simulink model "GPSReadLog"  (Simulink 6.6)
settings: Solver=FixedStepDiscrete  StartTime=0.0  StopTime=10.0  FixedStep=0.01  RelTol=1e-3
InitFcn:
  | initGPS
undefined symbols (not defined in the file or in its folder): gpsInit, gpsParse, gpsRead, gpsSeparate, logData, loggerInit, spiSend, u1, uartInit, y1
libraries: dsPICdrivers x15, simulink x1, xpclib x1
settings Model: Creator=ASL_Lab  LastModifiedBy=ASL_Lab  ProdHWDeviceType=16-bit Generic
settings OptimizationCC: InlineParams=on  OptimizeModelRefInitCode=on  LifeSpan=1
settings HardwareCC: ProdBitPerInt=16  ProdEndianess=LittleEndian  ProdWordSize=16  ProdHWDeviceType=16-bit Generic  TargetHWDeviceType=32-bit Generic
settings RTWCC: SystemTargetFile=dspic.tlc  TemplateMakefile=dspic_pic30_gcc.tmf  PostCodeGenCommand=dsPIC_Compile()  Description=Embedded Target for Microchip dsPIC (real-time)  GenerateReport=on  ProcessScript=dspic_make_rtw_hook  IncludeHyperlinkInReport=on  LaunchReport=on
settings RTWCC: CustomSource=|
  | clib\circBuffer.c
  | clib\gpsParse.c
  | clib\gpsSplit.c
  | clib\sbrk.c
  | clib\bufferedUART.c
  | clib\dataLogger.c
settings CodeAppCC: IgnoreCustomStorageClasses=off
settings STFCustomTargetCC: TargetFcnLib=ansi_tfl_tmw.mat  GenFloatMathFcnCalls=ANSI_C  ModelReferenceCompliant=off  IncludeMdlTerminateFcn=off  CombineOutputUpdateFcns=on  SuppressErrorStatus=on  ERTCustomFileBanners=on  SupportContinuousTime=off  SupportNonInlinedSFcns=off  SystemTargetFile=dspic.tlc
settings ERTTargetCC: TargetFcnLib=ansi_tfl_tmw.mat  GenFloatMathFcnCalls=ANSI_C  ModelReferenceCompliant=off  IncludeMdlTerminateFcn=off  SuppressErrorStatus=on  ModelStepFunctionPrototypeControlCompliant=off  ExtModeMexFile=noextcomm  InlinedParameterPlacement=NonHierarchical  ERTSrcFileBannerTemplate=dsPIC_code_template.cgt  ERTHdrFileBannerTemplate=dsPIC_code_template.cgt  ERTDataSrcFileTemplate=dsPIC_code_template.cgt  ERTDataHdrFileTemplate=dsPIC_code_template.cgt  ERTCustomFileTemplate=dsPIC_main.tlc
settings CustomProperty: DataType=string  Value=C:\PROGRA~1\MATLAB\R2007a\rtw\bin\win32\gmake

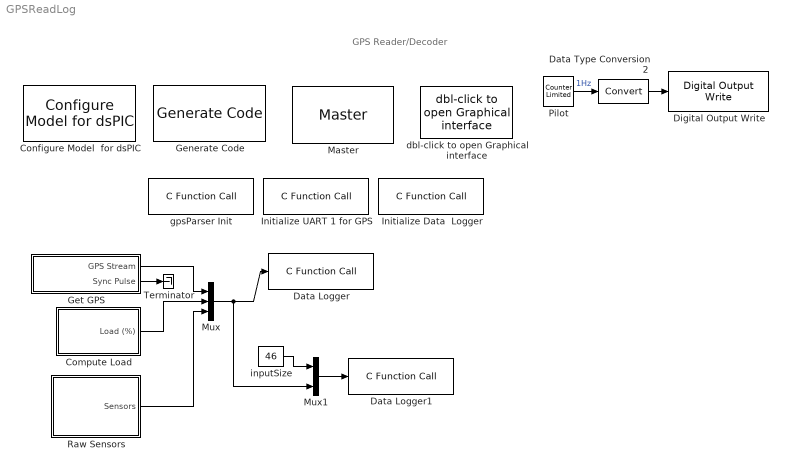
== system GPSReadLog ==
  note: GPS Reader/Decoder
  Compute Load : Subsystem
  Configure Model  for dsPIC : dsPICdrivers/Simulink Configuration/Configure Model  for dsPIC
  Data Logger : dsPICdrivers/OTHERS/C Function Call  Tag=dsPIC_dsPIC_CFunctionCall  fctName='logData'  INPUT_SIZE=46  INPUT1=uint8  INPUT2=--  INPUT3=--  OUTPUT_SIZE=1  OUTPUT1=--  SampleTime=-1  InputType=[ 2 ]  OutputType=[ ]  FctDeclaration=extern void logData(uint8_T* u1);  FctCall=logData(*%u1);  OrderingInOutPopup=None
  Data Logger1 : dsPICdrivers/OTHERS/C Function Call  Tag=dsPIC_dsPIC_CFunctionCall  fctName='spiSend'  INPUT_SIZE=47  INPUT1=uint8  INPUT2=--  INPUT3=--  OUTPUT_SIZE=1  OUTPUT1=--  SampleTime=-1  InputType=[ 2 ]  OutputType=[ ]  FctDeclaration=extern void spiSend(uint8_T* u1);  FctCall=spiSend(*%u1);  OrderingInOutPopup=None
  Data Type Conversion2 : DataTypeConversion  OutDataTypeMode=boolean
  Digital Output Write : dsPICdrivers/Digital I//O/Digital Output Write  Tag=dsPIC_Digital_Output  Priority=5  PORT=G  Pin=[ 14]  Simultaneous=off  OrderingInOutPopup=None
  Generate Code : dsPICdrivers/Simulink Configuration/Generate Code
  Get GPS : Subsystem
  Initialize Data  Logger : dsPICdrivers/OTHERS/C Function Call  Tag=dsPIC_dsPIC_CFunctionCall  fctName='loggerInit'  INPUT_SIZE=1  INPUT1=--  INPUT2=--  INPUT3=--  OUTPUT_SIZE=1  OUTPUT1=--  SampleTime=inf  InputType=[ ]  OutputType=[ ]  FctDeclaration=extern void loggerInit();  FctCall=loggerInit();  OrderingInOutPopup=None
  Initialize UART 1 for GPS : dsPICdrivers/OTHERS/C Function Call  Tag=dsPIC_dsPIC_CFunctionCall  fctName='uartInit'  INPUT_SIZE=1  INPUT1=--  INPUT2=--  INPUT3=--  OUTPUT_SIZE=1  OUTPUT1=--  SampleTime=inf  InputType=[ ]  OutputType=[ ]  FctDeclaration=extern void uartInit();  FctCall=uartInit();  OrderingInOutPopup=None
  Master : dsPICdrivers/Master  Tag=dsPIC_MASTER  Priority=1  TimeStepType=Timer1  picType=33fJ256MC710  fcy=40000000  Quartz_33f=12e6  PLLActive_33f=on  fcyDesired_33f=40e6  tmr1="[8  49999  0]"  tmr1Info="Time Step : 0.01  ;   Error : 0%  PR1=49999"  tmr2345="[0  0  0  0  0  0  0  0]"  tmr2345cfg=[-1 -1 -1 -1 -1 -1 -1 -1]  IOautoConf=on  typePort="[ 0   0   0   0   0   0   0   0   0   0   0   0   0   0   0   0   8   8   0   8   8   8   8   8   8   8   8   8   8   8   0   8   0   8   0   0   0   0   0   0   0   0   0   0   0   0   0   0   0   0   0   0   0   0   0   0   0   0   0   0   0   0   0   0   0   0   0   0   0   0   0   0   0   0   0   0   0   0   0   0   0   0   0   0   0   0   0   0   0   0   0   0   0   0   0   0   0   0   0   0   0   0   0   0   0   0   0   0   0   0  10   0 ]"  TRIS="[ 65535  65535  65535  65535  65535  65535  49151 ]"  ADPCFG=0  MasterBusyPort=None  MasterOverloadPort=None  FOSC=Quartz (XT - HS)  TempProtection_33f=TEMP_ON  FPBOR=<empty>  PWRT=disable  MCLR=<empty>  PowerSave=off
  Mux : Mux  Inputs=3
  Mux1 : Mux  Inputs=2
  Pilot : simulink/Sources/Counter Limited  SystemSampleTime=-1  uplimit=1  tsamp=1.0
  Raw Sensors : Subsystem
  Terminator : Terminator
  dbl-click to open Graphical interface : dsPICdrivers/Serial PORT/dbl-click to open Graphical interface  SystemSampleTime=-1  Nothing=0
  gpsParser Init : dsPICdrivers/OTHERS/C Function Call  Tag=dsPIC_dsPIC_CFunctionCall  fctName='gpsInit'  INPUT_SIZE=1  INPUT1=--  INPUT2=--  INPUT3=--  OUTPUT_SIZE=1  OUTPUT1=--  SampleTime=inf  InputType=[ ]  OutputType=[ ]  FctDeclaration=extern void gpsInit();  FctCall=gpsInit();  OrderingInOutPopup=None
  inputSize : Constant  Value=46  OutDataTypeMode=uint8
  wires:
  Pilot/1 -> Data Type Conversion2/1  "1Hz"
  Data Type Conversion2/1 -> Digital Output Write/1
  Get GPS/1(GPS Stream) -> Mux/1
  Mux/1 -> Data Logger/1, Mux1/2
  Compute Load/1(Load (%)) -> Mux/2
  Raw Sensors/1(Sensors) -> Mux/3
  Get GPS/2(Sync Pulse) -> Terminator/1
  Mux1/1 -> Data Logger1/1
  inputSize/1 -> Mux1/1

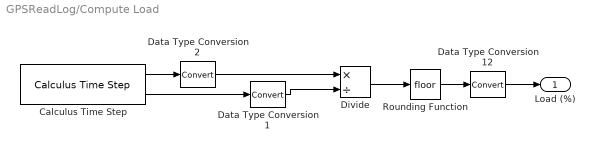
== system GPSReadLog/Compute Load ==
  Calculus Time Step : dsPICdrivers/OTHERS/Calculus Time Step  Tag=dsPIC_CalculusTimeStep  SampleTime=0.01  PR1chk=on
  Data Type Conversion1 : DataTypeConversion  OutDataTypeMode=single
  Data Type Conversion12 : DataTypeConversion  OutDataTypeMode=uint8
  Data Type Conversion2 : DataTypeConversion  OutDataTypeMode=single
  Divide : Product  Inputs=*/  OutDataTypeMode=double  OutScaling=2^-10
  Rounding Function : Rounding
  Load (%) : Outport
  wires:
  Calculus Time Step/1 -> Data Type Conversion2/1
  Calculus Time Step/2 -> Data Type Conversion1/1
  Divide/1 -> Rounding Function/1
  Rounding Function/1 -> Data Type Conversion12/1
  Data Type Conversion12/1 -> Load (%)/1
  Data Type Conversion1/1 -> Divide/2
  Data Type Conversion2/1 -> Divide/1

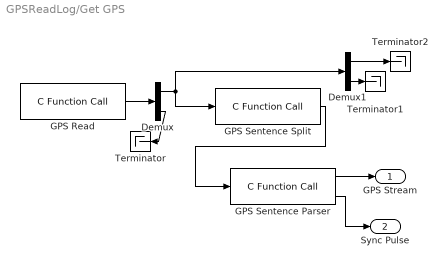
== system GPSReadLog/Get GPS ==
  Demux : Demux  Outputs=[25 1]
  Demux1 : Demux  Outputs=[1 24]
  GPS Read : dsPICdrivers/OTHERS/C Function Call  Tag=dsPIC_dsPIC_CFunctionCall  fctName='gpsRead'  INPUT_SIZE=1  INPUT1=--  INPUT2=--  INPUT3=--  OUTPUT_SIZE=26  OUTPUT1=uint8  SampleTime=-1  InputType=[ ]  OutputType=[ 2 ]  FctDeclaration=extern void gpsRead(uint8_T* y1);  FctCall=gpsRead(*%y1);  OrderingInOutPopup=None
  GPS Sentence Parser : dsPICdrivers/OTHERS/C Function Call  Tag=dsPIC_dsPIC_CFunctionCall  fctName='gpsParse'  INPUT_SIZE=127  INPUT1=uint8  INPUT2=--  INPUT3=--  OUTPUT_SIZE=27  OUTPUT1=uint8  SampleTime=-1  InputType=[ 2 ]  OutputType=[ 2 ]  FctDeclaration=extern void gpsParse(uint8_T* u1,uint8_T* y1);  FctCall=gpsParse(*%u1, *%y1);  OrderingInOutPopup=Output
  GPS Sentence Split : dsPICdrivers/OTHERS/C Function Call  Tag=dsPIC_dsPIC_CFunctionCall  fctName='gpsSeparate'  INPUT_SIZE=25  INPUT1=uint8  INPUT2=--  INPUT3=--  OUTPUT_SIZE=127  OUTPUT1=uint8  SampleTime=-1  InputType=[ 2 ]  OutputType=[ 2 ]  FctDeclaration=extern void gpsSeparate(uint8_T* u1,uint8_T* y1);  FctCall=gpsSeparate(*%u1, *%y1);  OrderingInOutPopup=None
  Terminator : Terminator
  Terminator1 : Terminator
  Terminator2 : Terminator
  GPS Stream : Outport
  Sync Pulse : Outport  Port=2
  wires:
  GPS Sentence Split/1 -> GPS Sentence Parser/1
  GPS Read/1 -> Demux/1
  Demux/1 -> GPS Sentence Split/1, Demux1/1
  Demux/2 -> Terminator/1
  Demux1/2 -> Terminator1/1
  Demux1/1 -> Terminator2/1
  GPS Sentence Parser/1 -> GPS Stream/1
  GPS Sentence Parser/2 -> Sync Pulse/1

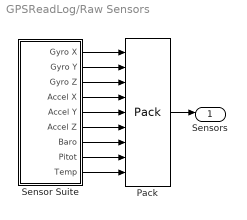
== system GPSReadLog/Raw Sensors ==
  Pack : xpclib/UDP/Pack  datatypes={'uint16', 'uint16', 'uint16', 'uint16', 'uint16', 'uint16', 'uint16', 'uint16', 'uint16',}  byteAlign=1
  Sensor Suite : Subsystem
  Sensors : Outport
  wires:
  Sensor Suite/1(Gyro X) -> Pack/1
  Sensor Suite/2(Gyro Y) -> Pack/2
  Sensor Suite/3(Gyro Z) -> Pack/3
  Sensor Suite/4(Accel X) -> Pack/4
  Sensor Suite/5(Accel Y) -> Pack/5
  Sensor Suite/6(Accel Z) -> Pack/6
  Sensor Suite/7(Baro) -> Pack/7
  Sensor Suite/8(Pitot) -> Pack/8
  Sensor Suite/9(Temp) -> Pack/9
  Pack/1 -> Sensors/1

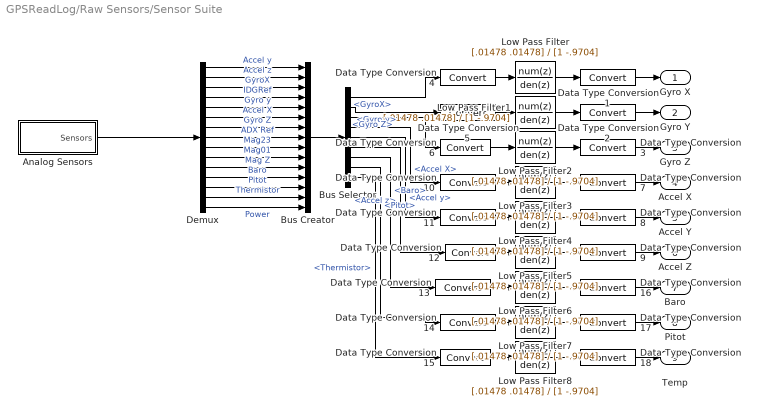
== system GPSReadLog/Raw Sensors/Sensor Suite ==
  Analog Sensors : Subsystem
  Bus Creator : BusCreator  Inputs=15
  Bus Selector : BusSelector  OutputSignals=GyroX,Gyro y,Gyro Z,Accel X,Accel y,Accel z,Baro,Pitot,Thermistor
  Data Type Conversion{1..3,7..9,16..18} (9 alike) : DataTypeConversion  OutDataTypeMode=uint16
  Data Type Conversion{4..6,10..15} (9 alike) : DataTypeConversion  OutDataTypeMode=double
  Demux : Demux  Outputs=15
  Low Pass Filter{,1..8} (9 alike) : DiscreteTransferFcn  Numerator=[.01478 .01478]  Denominator=[1 -.9704]  SampleTime=.01
  Gyro X : Outport
  Gyro Y : Outport  Port=2
  Gyro Z : Outport  Port=3
  Accel X : Outport  Port=4
  Accel Y : Outport  Port=5
  Accel Z : Outport  Port=6
  Baro : Outport  Port=7
  Pitot : Outport  Port=8
  Temp : Outport  Port=9
  wires:
  Demux/1 -> Bus Creator/1  "Accel y"
  Demux/2 -> Bus Creator/2  "Accel z"
  Demux/3 -> Bus Creator/3  "GyroX"
  Demux/4 -> Bus Creator/4  "IDGRef"
  Demux/5 -> Bus Creator/5  "Gyro y"
  Demux/6 -> Bus Creator/6  "Accel X"
  Demux/7 -> Bus Creator/7  "Gyro Z"
  Demux/8 -> Bus Creator/8  "ADX Ref"
  Demux/9 -> Bus Creator/9  "Mag23"
  Demux/10 -> Bus Creator/10  "Mag01"
  Demux/11 -> Bus Creator/11  "Mag Z"
  Demux/12 -> Bus Creator/12  "Baro"
  Demux/13 -> Bus Creator/13  "Pitot"
  Demux/14 -> Bus Creator/14  "Thermistor"
  Demux/15 -> Bus Creator/15  "Power"
  Bus Creator/1 -> Bus Selector/1
  Bus Selector/1 -> Data Type Conversion4/1  "<GyroX>"
  Bus Selector/2 -> Data Type Conversion5/1  "<Gyro y>"
  Bus Selector/3 -> Data Type Conversion6/1  "<Gyro Z>"
  Low Pass Filter/1 -> Data Type Conversion1/1
  Low Pass Filter1/1 -> Data Type Conversion2/1
  Data Type Conversion4/1 -> Low Pass Filter/1
  Data Type Conversion5/1 -> Low Pass Filter1/1
  Analog Sensors/1(Sensors) -> Demux/1
  Data Type Conversion6/1 -> Low Pass Filter2/1
  Low Pass Filter2/1 -> Data Type Conversion3/1
  Low Pass Filter3/1 -> Data Type Conversion7/1
  Low Pass Filter4/1 -> Data Type Conversion8/1
  Data Type Conversion10/1 -> Low Pass Filter3/1
  Data Type Conversion11/1 -> Low Pass Filter4/1
  Data Type Conversion12/1 -> Low Pass Filter5/1
  Low Pass Filter5/1 -> Data Type Conversion9/1
  Bus Selector/4 -> Data Type Conversion10/1  "<Accel X>"
  Bus Selector/5 -> Data Type Conversion11/1  "<Accel y>"
  Bus Selector/6 -> Data Type Conversion12/1  "<Accel z>"
  Low Pass Filter7/1 -> Data Type Conversion17/1
  Data Type Conversion14/1 -> Low Pass Filter7/1
  Data Type Conversion15/1 -> Low Pass Filter8/1
  Low Pass Filter8/1 -> Data Type Conversion18/1
  Bus Selector/7 -> Data Type Conversion13/1  "<Baro>"
  Bus Selector/8 -> Data Type Conversion14/1  "<Pitot>"
  Bus Selector/9 -> Data Type Conversion15/1  "<Thermistor>"
  Data Type Conversion13/1 -> Low Pass Filter6/1
  Low Pass Filter6/1 -> Data Type Conversion16/1
  Data Type Conversion1/1 -> Gyro X/1
  Data Type Conversion2/1 -> Gyro Y/1
  Data Type Conversion3/1 -> Gyro Z/1
  Data Type Conversion7/1 -> Accel X/1
  Data Type Conversion8/1 -> Accel Y/1
  Data Type Conversion9/1 -> Accel Z/1
  Data Type Conversion16/1 -> Baro/1
  Data Type Conversion17/1 -> Pitot/1
  Data Type Conversion18/1 -> Temp/1

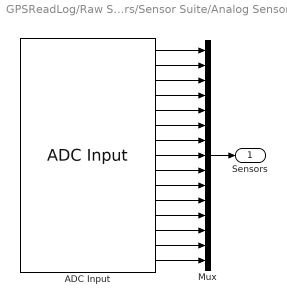
== system GPSReadLog/Raw Sensors/Sensor Suite/Analog Sensors ==
  ADC Input : dsPICdrivers/Peripheral I//O/ADC Input  Tag=dsPIC_ADC  Priority=5  ADC_TYPE=12 bits  ADC_MODE=Continuous sampling & get last channel value  NbrSampleStep=1  VoltRefpopup="AVdd  -  AVss"  OutFormatBitspopup=0000 dddd dddd dddd : Integer  InterruptPriority=6  ANCHANNELS=[0 1 3 4 5 6 7 8 9 10 11 12 13 15 16]  MaxName=ANmax = 4096  Rin=1e2  ADCS=53  SAMC=1  Temperature=25  DMAChannel=1  SampleTime=.01  Status="OK  |  Tsmp=6.750e-007 |  T/Channel=1.012e-005 |  Tall=1.519e-004"
  Mux : Mux  Inputs=15
  Sensors : Outport
  wires:
  ADC Input/1 -> Mux/1
  ADC Input/2 -> Mux/2
  ADC Input/3 -> Mux/3
  ADC Input/4 -> Mux/4
  ADC Input/5 -> Mux/5
  ADC Input/6 -> Mux/6
  ADC Input/7 -> Mux/7
  ADC Input/8 -> Mux/8
  ADC Input/9 -> Mux/9
  ADC Input/10 -> Mux/10
  ADC Input/11 -> Mux/11
  ADC Input/12 -> Mux/12
  ADC Input/13 -> Mux/13
  ADC Input/14 -> Mux/14
  ADC Input/15 -> Mux/15
  Mux/1 -> Sensors/1
